simulink model "Simulacion"  (R2022a)
settings: Solver=VariableStepAuto  StartTime=0.0  StopTime=1  RelTol=1e-3
values from neighbouring files (symbols this model uses):
  Cbus = 80e-3    (= 0.08)    [Simulacion.m]
  D = 1e-3    (= 0.001)    [Simulacion.m]
  f = 50    [Simulacion.m]
  Fs = Vs*sqrt(2/3)/(2*pi*f)    [Simulacion.m]
  fsw = 4e3    (= 4000)    [Simulacion.m]
  J = 127    [Simulacion.m]
  ki_id = (wni^2)*Lr*sigma    (= 491.599501999)    [Simulacion.m]
  ki_idg = (wnig^2)*Lg    (= 56.8489213503)    [Simulacion.m]
  ki_iq = ki_id    (= 491.599501999)    [Simulacion.m]
  ki_iqg = ki_idg    (= 56.8489213503)    [Simulacion.m]
  ki_n = ((wnn^2)*J)/p    (= 25400)    [Simulacion.m]
  ki_v = -300000    [Simulacion.m]
  kp_id = (2*wni*sigma*Lr)-Rr    (= 0.5771)    [Simulacion.m]
  kp_idg = (2*wnig*Lg)-Rg    (= 0.301572894745)    [Simulacion.m]
  kp_iq = kp_id    (= 0.5771)    [Simulacion.m]
  kp_iqg = kp_idg    (= 0.301572894745)    [Simulacion.m]
  kp_n = (2*wnn*J)/p    (= 2540)    [Simulacion.m]
  kp_v = -1000    [Simulacion.m]
  Kpg = 1/(1.5*Vs*sqrt(2/3))    [Simulacion.m]
  Kqg = -Kpg    [Simulacion.m]
  Lg = 400e-6    (= 0.0004)    [Simulacion.m]
  Lm = 2.5e-3    (= 0.0025)    [Simulacion.m]
  Ls = Lm+Lsi    (= 0.002587)    [Simulacion.m]
  Lsi = 0.087e-3    (= 8.7e-05)    [Simulacion.m]
  p = 2    [Simulacion.m]
  Ps = 2e6    (= 2000000)    [Simulacion.m]
  Rg = 20e-6    (= 2e-05)    [Simulacion.m]
  Rr = 2.9e-3    (= 0.0029)    [Simulacion.m]
  Rs = 2.6e-3    (= 0.0026)    [Simulacion.m]
  Tem = 12732    [Simulacion.m]
  Ts = 1/fsw/50    (= 5e-06)    [Simulacion.m]
  Vbus = Vr_stator*sqrt(2)    [Simulacion.m]
  Vs = 690    [Simulacion.m]
undefined symbols (not defined in the file or in its folder): DiscIntNeverNeededParam
libraries: spsSeriesRLCBranchLib x4, spsThreePhaseVIMeasurementLib x3, spsPWMGenerator2LevelLib x2, spsUniversalBridgeLib x2, spsAsynchronousMachineSIUnitsLib x1, spsGroundLib x1, spsThreePhaseProgrammableVoltageSourceLib x1, spsThreePhaseTransformerTwoWindingsLib x1, spsVoltageMeasurementLib x1, spspowerguiLib x1
settings Model: Creator=ontib  LastModifiedBy=ontib

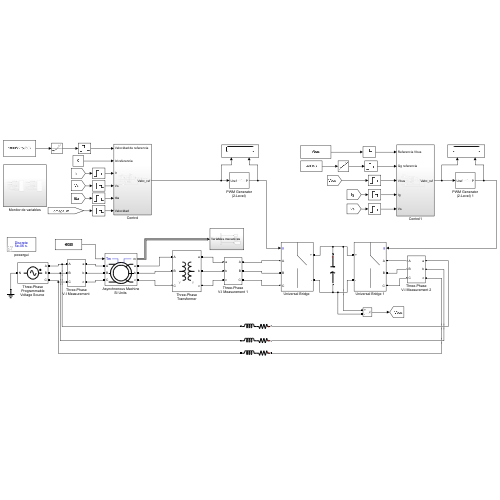
[thumbnail: Simulink's stored preview of the top-level diagram]
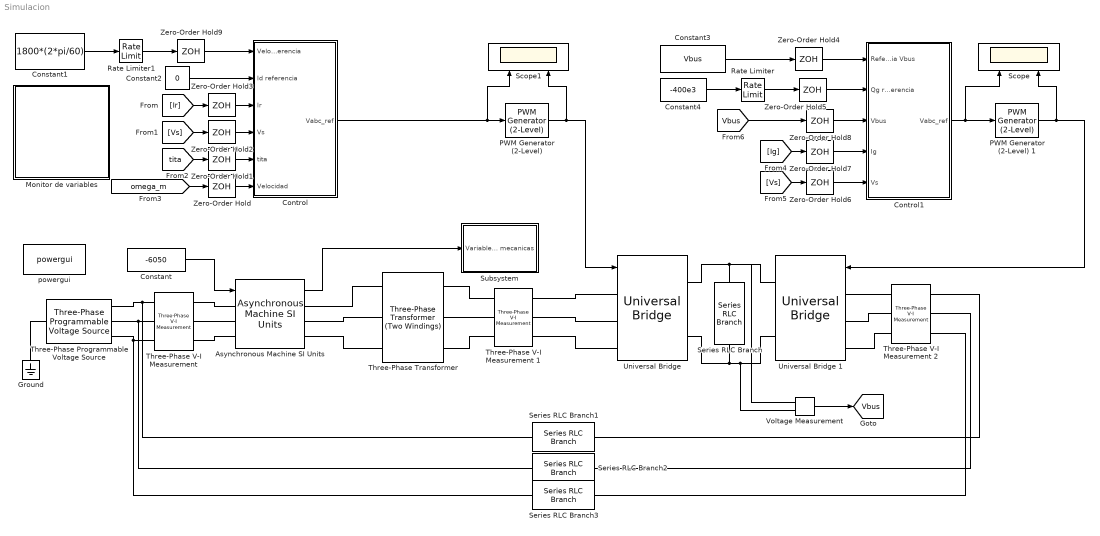
== system Simulacion ==
  "Asynchronous Machine SI Units " : spsAsynchronousMachineSIUnitsLib/Asynchronous Machine SI Units  RotorType=Wound  PresetModel=No  MechanicalLoad=Torque Tm  ShowDetailedParameters=on  ReferenceFrame=Rotor  Units=SI  MeasurementBus=off  NominalParameters=[Ps Vs f]  VoltageRatio=1  Stator=[Rs Ls]  Rotor=[Rr Lsi]  Cage1=[0.4155 0.002066]  Cage2=[0.4168 0.0003495]  Lm=Lm  Mechanical=[J D 2]  PolePairs=2  InitialConditions=[1 0 0 0 0 0 0 0]  SimulateSaturation=off  Saturation=[14.03593122, 27.81365428, 53.79336849, 72.68890987, 97.98006896, 148.6815601, 215.7428561, 302.9841135, 428.7778367 ; 230, 322, 414, 460, 506, 552, 598, 644, 690]  LoadFlowParameters=1492000  TsPowergui=0  TsBlock=-1  IterativeModel=Trapezoidal non iterative  IterativeDiscreteModel=Trapezoidal non iterative  Pmec=1.492e+006
  Constant : Constant  Value=-6050
  Constant1 : Constant  Value=1800*(2*pi/60)
  Constant2 : Constant  Value=0
  Constant3 : Constant  Value=Vbus
  Constant4 : Constant  Value=-400e3
  Control : Subsystem
  Control1 : Subsystem
  Ground : spsGroundLib/Ground  LConnTagsString=a
  Monitor de variables : Subsystem
  "PWM Generator (2-Level) " : spsPWMGenerator2LevelLib/PWM Generator (2-Level)  ModulatorType=Three-phase bridge (6 pulses)  ModulatorMode=Unsynchronized  Fc=fsw  Pc=0  nF=27  MinMax="[ -1  1 ]"  SamplingTechnique=Symmetrical regular (single edge)  ModulatingSignals=off  m=0.8  Freq=60  Phase=0  Ts=0  ShowCarrierOutport=off
  PWM Generator (2-Level) 1 : spsPWMGenerator2LevelLib/PWM Generator (2-Level)  ModulatorType=Three-phase bridge (6 pulses)  ModulatorMode=Unsynchronized  Fc=fsw  Pc=0  nF=27  MinMax="[ -1  1 ]"  SamplingTechnique=Symmetrical regular (single edge)  ModulatingSignals=off  m=0.8  Freq=60  Phase=0  Ts=0  ShowCarrierOutport=off
  Rate Limiter : RateLimiter  RisingSlewLimit=1000e3/2  FallingSlewLimit=-1000e3/2  SampleTimeMode=inherited
  Rate Limiter1 : RateLimiter  RisingSlewLimit=100  FallingSlewLimit=-100  SampleTimeMode=inherited
  Scope : Scope  NumInputPorts=2
  Scope1 : Scope  NumInputPorts=2
  Series RLC Branch : spsSeriesRLCBranchLib/Series RLC Branch  LConnTagsString=__new0  RConnTagsString=__new0  BranchType=C  Resistance=1  Inductance=1e-3  SetiL0=off  InitialCurrent=0  Capacitance=Cbus  Setx0=off  InitialVoltage=0  Measurements=Branch voltage
  Series RLC Branch1 : spsSeriesRLCBranchLib/Series RLC Branch  LConnTagsString=__new0  RConnTagsString=__new0  BranchType=RL  Resistance=Rg  Inductance=Lg  SetiL0=off  InitialCurrent=0  Capacitance=Cbus  Setx0=off  InitialVoltage=0  Measurements=Branch voltage
  Series RLC Branch2 : spsSeriesRLCBranchLib/Series RLC Branch  LConnTagsString=__new0  RConnTagsString=__new0  BranchType=RL  Resistance=Rg  Inductance=Lg  SetiL0=off  InitialCurrent=0  Capacitance=Cbus  Setx0=off  InitialVoltage=0  Measurements=Branch voltage
  Series RLC Branch3 : spsSeriesRLCBranchLib/Series RLC Branch  LConnTagsString=__new0  RConnTagsString=__new0  BranchType=RL  Resistance=Rg  Inductance=Lg  SetiL0=off  InitialCurrent=0  Capacitance=Cbus  Setx0=off  InitialVoltage=0  Measurements=Branch voltage
  Subsystem : Subsystem
  "Three-Phase Programmable Voltage Source " : spsThreePhaseProgrammableVoltageSourceLib/Three-Phase Programmable Voltage Source  PositiveSequence="[Vs  0 f]"  VariationEntity=None  VariationType=Table of time-amplitude pairs  VariationTypeAlt=Step  VariationStep=0.5  VariationRate=10  VariationMagnitude=0.3  VariationFrequency=2  VariationTiming=[1 2]  VariationPhaseA=off  Amplitudes=[1 0.8 1.2 1.0]  TimeValues=[0 0.1 0.15 0.2]  HarmonicGeneration=off  HarmonicA=[3 0.2 -25 0]  HarmonicB=[2 0.15 35 2]  Timing="[0.05  3]"  BusType=swing  Pref=0  Qref=0  Qmin=-inf  Qmax=inf
  Three-Phase Transformer : spsThreePhaseTransformerTwoWindingsLib/Three-Phase Transformer (Two Windings)  Winding1Connection=Y  Winding2Connection=Y  CoreType=Three single-phase transformers  SetSaturation=off  Hysteresis=off  DataFile='hysteresis'  SetInitialFlux=off  Measurements=None  UNITS=SI  NominalPower=[ Ps , f ]  Winding1=[Vs 0 0]  Winding2=[Vs/u 0 0]  Rm=1.0804e+06  Lm=3439.2  L0=0.5  Saturation=[0 0;0.66653 2292.3;277.72 2903.6]  InitialFluxes=[ 0.8 , -0.8 , 0.7 ]  BreakLoop=off  DiscreteSolver=Trapezoidal iterative  DataType=on  TransfoNumber=1
  "Three-Phase V-I Measurement " : spsThreePhaseVIMeasurementLib/Three-Phase V-I Measurement  VoltageMeasurement=phase-to-ground  SetLabelV=on  LabelV=Vs  Vpu=off  VpuLL=off  CurrentMeasurement=yes  SetLabelI=on  LabelI=Is  Ipu=off  Pbase=100e6  Vbase=500e3  OutputType=Complex  PhasorSimulation=off  PSBequivalent=0
  Three-Phase V-I Measurement 1 : spsThreePhaseVIMeasurementLib/Three-Phase V-I Measurement  VoltageMeasurement=no  SetLabelV=off  LabelV=Vs  Vpu=off  VpuLL=off  CurrentMeasurement=yes  SetLabelI=on  LabelI=Ir  Ipu=off  Pbase=100e6  Vbase=500e3  OutputType=Complex  PhasorSimulation=off  PSBequivalent=0
  Three-Phase V-I Measurement 2 : spsThreePhaseVIMeasurementLib/Three-Phase V-I Measurement  VoltageMeasurement=no  SetLabelV=off  LabelV=Vs  Vpu=off  VpuLL=off  CurrentMeasurement=yes  SetLabelI=on  LabelI=Ig  Ipu=off  Pbase=100e6  Vbase=500e3  OutputType=Complex  PhasorSimulation=off  PSBequivalent=0
  "Universal Bridge " : spsUniversalBridgeLib/Universal Bridge  Arms=3  SnubberResistance=1e5  SnubberCapacitance=inf  Device=Ideal Switches  Ron=1e-3  Lon=0  ForwardVoltages="[  0  0  ]"  ForwardVoltage=0  GTOparameters=[ 10e-6 , 20e-6 ]  IGBTparameters=[ 1e-6 , 2e-6 ]  Measurements=None  Measurements_2=None  converterType=Rectifier
  Universal Bridge 1 : spsUniversalBridgeLib/Universal Bridge  Arms=3  SnubberResistance=1e5  SnubberCapacitance=inf  Device=Ideal Switches  Ron=1e-3  Lon=0  ForwardVoltages="[  0  0  ]"  ForwardVoltage=0  GTOparameters=[ 10e-6 , 20e-6 ]  IGBTparameters=[ 1e-6 , 2e-6 ]  Measurements=None  Measurements_2=None  converterType=Rectifier
  Voltage Measurement : spsVoltageMeasurementLib/Voltage Measurement  PhasorSimulation=off  OutputType=Complex  PSBequivalent=0
  Zero-Order Hold{,1..9} (10 alike) : ZeroOrderHold  SampleTime=1/fsw
  powergui : spspowerguiLib/powergui  Priority=1  SimulationMode=Discrete  SampleTime=Ts  frequency=60  Iterations=50  frequencyindice=50  Pbase=100e6  ErrMax=1e-4  UnitsV=kV  UnitsW=MW  buscounter=0  FunctionMessages=off  echomessages=off  EnableUseOfTLC=off  CurrentSourceSwitches=off  DisableSnubberDevices=off  DisableRonSwitches=off  DisableVfSwitches=off  DisplayEquations=off  AutomaticDiscreteSolvers=off  SolverType=Tustin/Backward Euler (TBE)  Interpol=off  ExternalGateDelay=off  methode=off  Ts=100  x0status=blocks  SPID=on  SwTol=0  HookPort=off  NonlinearTolerance=1e-4  nMaxIteration=100  ContinueOnMaxIteration=off  RestoreLinks=warning  ResistiveCurrentMeasurement=off  Frange=[0:2:500]  Ylog=off  Xlog=on  ShowGrid=off  save=off  variable=ZData  structure=0  ZoomFFT=off  StartTime=0.0  cycles=1  DisplayStyle=1  fundamental=60  FreqAxis=off  MaxFrequency=1000  frequencyindicesteady=1  RmsSteady=1  display=off
  tag scope: Vbus=global
  wires:
  "PWM Generator (2-Level) "/1 -> "Universal Bridge "/1, Scope1/2
  Control/1(Vabc_ref) -> Scope1/1, "PWM Generator (2-Level) "/1
  [Ir] -> Zero-Order Hold3/1
  [Vs] -> Zero-Order Hold2/1
  Constant2/1 -> Control/2(Id referencia)
  Zero-Order Hold9/1 -> Control/1(Velocidad de referencia)
  "Asynchronous Machine SI Units "/1 -> Subsystem/1(Variables mecanicas)
  [tita] -> Zero-Order Hold1/1
  [omega_m] -> Zero-Order Hold/1
  Constant/1 -> "Asynchronous Machine SI Units "/1
  Zero-Order Hold/1 -> Control/6(Velocidad)
  Zero-Order Hold1/1 -> Control/5(tita)
  Zero-Order Hold2/1 -> Control/4(Vs)
  Zero-Order Hold3/1 -> Control/3(Ir)
  PWM Generator (2-Level) 1/1 -> Universal Bridge 1/1, Scope/2
  Zero-Order Hold7/1 -> Control1/4(Ig)
  Zero-Order Hold6/1 -> Control1/5(Vs)
  [Ig] -> Zero-Order Hold7/1
  Constant4/1 -> Rate Limiter/1
  [Vs] -> Zero-Order Hold6/1
  Control1/1(Vabc_ref) -> Scope/1, PWM Generator (2-Level) 1/1
  Constant3/1 -> Zero-Order Hold4/1
  Zero-Order Hold4/1 -> Control1/1(Referencia Vbus)
  Rate Limiter/1 -> Zero-Order Hold5/1
  Zero-Order Hold5/1 -> Control1/2(Qg referencia)
  Voltage Measurement/1 -> [Vbus]
  [Vbus] -> Zero-Order Hold8/1
  Zero-Order Hold8/1 -> Control1/3(Vbus)
  Constant1/1 -> Rate Limiter1/1
  Rate Limiter1/1 -> Zero-Order Hold9/1
  connections:
  Ground/LConn1 -- "Three-Phase Programmable Voltage Source "/LConn1
  "Three-Phase V-I Measurement "/RConn1 -- "Asynchronous Machine SI Units "/LConn1
  "Asynchronous Machine SI Units "/LConn2 -- "Three-Phase V-I Measurement "/RConn2
  "Three-Phase V-I Measurement "/RConn3 -- "Asynchronous Machine SI Units "/LConn3
  "Three-Phase V-I Measurement "/LConn1 -- Series RLC Branch1/RConn1 -- "Three-Phase Programmable Voltage Source "/RConn1
  "Three-Phase V-I Measurement "/LConn2 -- Series RLC Branch2/RConn1 -- "Three-Phase Programmable Voltage Source "/RConn2
  "Three-Phase V-I Measurement "/LConn3 -- Series RLC Branch3/RConn1 -- "Three-Phase Programmable Voltage Source "/RConn3
  Three-Phase V-I Measurement 1/LConn1 -- "Universal Bridge "/LConn1
  Three-Phase V-I Measurement 1/LConn2 -- "Universal Bridge "/LConn2
  Three-Phase V-I Measurement 1/LConn3 -- "Universal Bridge "/LConn3
  Series RLC Branch/LConn1 -- Voltage Measurement/LConn1 -- Universal Bridge 1/RConn1 -- "Universal Bridge "/RConn1
  Universal Bridge 1/RConn2 -- Voltage Measurement/LConn2 -- "Universal Bridge "/RConn2 -- Series RLC Branch/RConn1
  Three-Phase V-I Measurement 2/LConn1 -- Universal Bridge 1/LConn1
  Three-Phase V-I Measurement 2/LConn2 -- Universal Bridge 1/LConn2
  Three-Phase V-I Measurement 2/LConn3 -- Universal Bridge 1/LConn3
  Series RLC Branch1/LConn1 -- Three-Phase V-I Measurement 2/RConn1
  Series RLC Branch2/LConn1 -- Three-Phase V-I Measurement 2/RConn2
  Series RLC Branch3/LConn1 -- Three-Phase V-I Measurement 2/RConn3
  Three-Phase Transformer/RConn1 -- Three-Phase V-I Measurement 1/RConn1
  Three-Phase V-I Measurement 1/RConn2 -- Three-Phase Transformer/RConn2
  Three-Phase V-I Measurement 1/RConn3 -- Three-Phase Transformer/RConn3
  Three-Phase Transformer/LConn1 -- "Asynchronous Machine SI Units "/RConn1
  Three-Phase Transformer/LConn2 -- "Asynchronous Machine SI Units "/RConn2
  "Asynchronous Machine SI Units "/RConn3 -- Three-Phase Transformer/LConn3

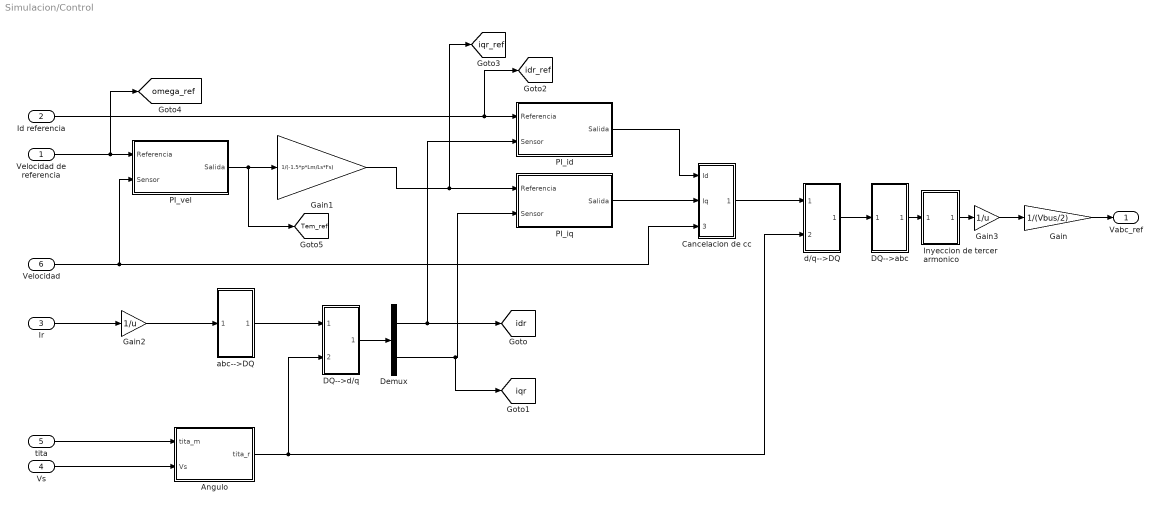
== system Simulacion/Control ==
  Velocidad de referencia : Inport
  Id referencia : Inport  Port=2
  Ir : Inport  Port=3
  Vs : Inport  Port=4
  tita : Inport  Port=5
  Velocidad : Inport  Port=6
  Angulo : Subsystem
  Cancelacion de cc : Subsystem
  DQ-->abc : Subsystem
  DQ-->d/q : Subsystem
  Demux : Demux  Outputs=2
  Gain : Gain  Gain=1/(Vbus/2)
  Gain1 : Gain  Gain=1/(-1.5*p*Lm/Ls*Fs)
  Gain2 : Gain  Gain=1/u
  Gain3 : Gain  Gain=1/u
  Inyeccion de tercer armonico : Subsystem
  PI_id : Subsystem
  PI_iq : Subsystem
  PI_vel : Subsystem
  abc-->DQ : Subsystem
  d/q-->DQ : Subsystem
  Vabc_ref : Outport
  tag scope: Tem_ref=global, idr=global, idr_ref=global, iqr=global, iqr_ref=global, omega_ref=global
  wires:
  Gain/1 -> Vabc_ref/1
  d/q-->DQ/1(DQ) -> DQ-->abc/1(D/Q)
  abc-->DQ/1(D/Q) -> DQ-->d/q/1(D/Q)
  Ir/1 -> Gain2/1
  DQ-->abc/1(abc) -> Inyeccion de tercer armonico/1(abc)
  Inyeccion de tercer armonico/1(Out1) -> Gain3/1
  tita/1 -> Angulo/1(tita_m)
  Vs/1 -> Angulo/2(Vs)
  Angulo/1(tita_r) -> DQ-->d/q/2(tita), d/q-->DQ/2(tita)
  Cancelacion de cc/1(d/q) -> d/q-->DQ/1(d/q)
  PI_iq/1(Salida) -> Cancelacion de cc/2(Iq)
  PI_id/1(Salida) -> Cancelacion de cc/1(Id)
  Velocidad/1 -> PI_vel/2(Sensor), Cancelacion de cc/3(omega)
  DQ-->d/q/1(d/q) -> Demux/1
  Demux/2 -> [iqr], PI_iq/2(Sensor)
  Demux/1 -> [idr], PI_id/2(Sensor)
  Velocidad de referencia/1 -> [omega_ref], PI_vel/1(Referencia)
  PI_vel/1(Salida) -> [Tem_ref], Gain1/1
  Gain1/1 -> [iqr_ref], PI_iq/1(Referencia)
  Id referencia/1 -> [idr_ref], PI_id/1(Referencia)
  Gain3/1 -> Gain/1
  Gain2/1 -> abc-->DQ/1(abc)

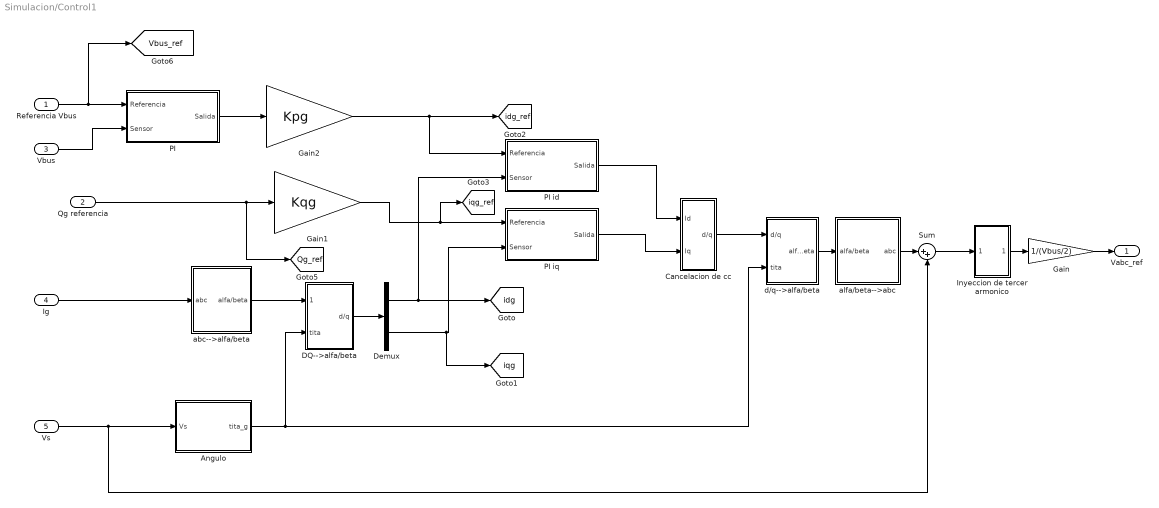
== system Simulacion/Control1 ==
  Referencia Vbus : Inport
  Qg referencia : Inport  Port=2
  Vbus : Inport  Port=3
  Ig : Inport  Port=4
  Vs : Inport  Port=5
  Angulo : Subsystem
  Cancelacion de cc : Subsystem
  DQ-->alfa/beta : Subsystem
  Demux : Demux  Outputs=2
  Gain : Gain  Gain=1/(Vbus/2)
  Gain1 : Gain  Gain=Kqg
  Gain2 : Gain  Gain=Kpg
  Inyeccion de tercer armonico : Subsystem
  PI : Subsystem
  PI id : Subsystem
  PI iq : Subsystem
  Sum : Sum  Inputs=|++
  abc-->alfa/beta : Subsystem
  alfa/beta-->abc : Subsystem
  d/q-->alfa/beta : Subsystem
  Vabc_ref : Outport
  tag scope: Qg_ref=global, Vbus_ref=global, idg=global, idg_ref=global, iqg=global, iqg_ref=global
  wires:
  Gain/1 -> Vabc_ref/1
  d/q-->alfa/beta/1(alfa/beta) -> alfa/beta-->abc/1(alfa/beta)
  abc-->alfa/beta/1(alfa/beta) -> DQ-->alfa/beta/1(alfa/beta)
  Ig/1 -> abc-->alfa/beta/1(abc)
  Inyeccion de tercer armonico/1(Out1) -> Gain/1
  Vs/1 -> Sum/2, Angulo/1(Vs)
  Angulo/1(tita_g) -> d/q-->alfa/beta/2(tita), DQ-->alfa/beta/2(tita)
  Cancelacion de cc/1(d/q) -> d/q-->alfa/beta/1(d/q)
  PI iq/1(Salida) -> Cancelacion de cc/2(Iq)
  PI id/1(Salida) -> Cancelacion de cc/1(Id)
  DQ-->alfa/beta/1(d/q) -> Demux/1
  Demux/2 -> [iqg], PI iq/2(Sensor)
  Demux/1 -> [idg], PI id/2(Sensor)
  Qg referencia/1 -> [Qg_ref], Gain1/1
  Gain1/1 -> [iqg_ref], PI iq/1(Referencia)
  PI/1(Salida) -> Gain2/1
  Gain2/1 -> [idg_ref], PI id/1(Referencia)
  Referencia Vbus/1 -> [Vbus_ref], PI/1(Referencia)
  Vbus/1 -> PI/2(Sensor)
  alfa/beta-->abc/1(abc) -> Sum/1
  Sum/1 -> Inyeccion de tercer armonico/1(abc)

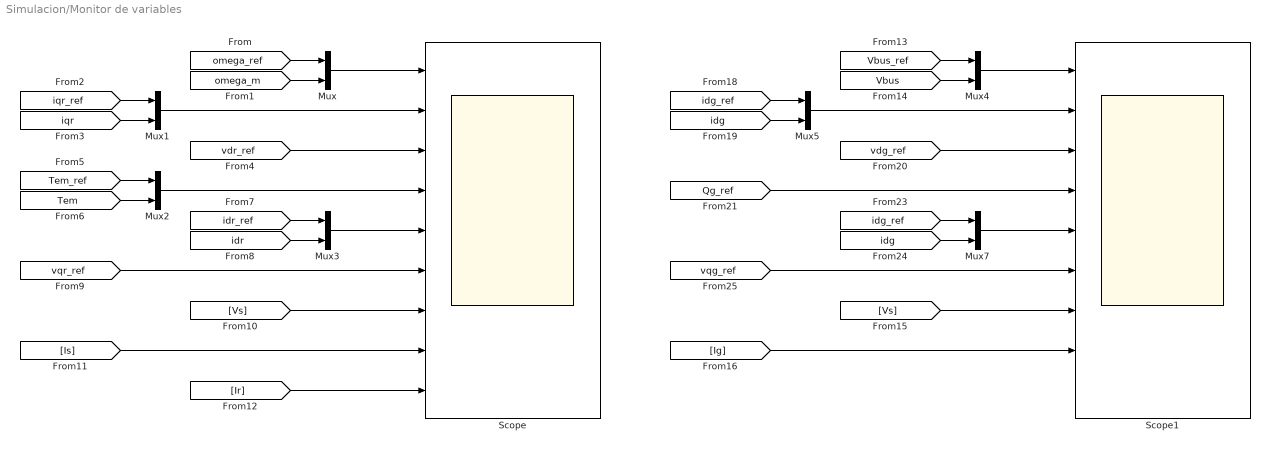
== system Simulacion/Monitor de variables ==
  Mux{,1..5,7} (7 alike) : Mux  Inputs=2
  Scope : Scope  NumInputPorts=9
  Scope1 : Scope  NumInputPorts=9
  wires:
  [omega_ref] -> Mux/1
  [omega_m] -> Mux/2
  [iqr_ref] -> Mux1/1
  [iqr] -> Mux1/2
  Mux/1 -> Scope/1
  Mux1/1 -> Scope/2
  [vdr_ref] -> Scope/3
  Mux2/1 -> Scope/4
  [Tem_ref] -> Mux2/1
  [Tem] -> Mux2/2
  [idr_ref] -> Mux3/1
  [idr] -> Mux3/2
  Mux3/1 -> Scope/5
  [vqr_ref] -> Scope/6
  [Vs] -> Scope/7
  [Ir] -> Scope/9
  [Is] -> Scope/8
  [idg] -> Mux7/2
  Mux7/1 -> Scope1/5
  [Ig] -> Scope1/8
  [Vbus_ref] -> Mux4/1
  [Vbus] -> Mux4/2
  [idg_ref] -> Mux7/1
  [vqg_ref] -> Scope1/6
  Mux4/1 -> Scope1/1
  Mux5/1 -> Scope1/2
  [vdg_ref] -> Scope1/3
  [idg] -> Mux5/2
  [idg_ref] -> Mux5/1
  [Vs] -> Scope1/7
  [Qg_ref] -> Scope1/4

== system Simulacion/Subsystem ==
  Variables mecanicas : Inport
  Bus Selector : BusSelector  OutputSignals=Mechanical.Rotor angle thetam (rad),Mechanical.Electromagnetic torque Te (N*m),Mechanical.Rotor speed (wm)
  tag scope: Tem=global, omega_m=global, tita=global
  wires:
  Bus Selector/1 -> [tita]  "<Rotor angle thetam (rad)>"
  Variables mecanicas/1 -> Bus Selector/1
  Bus Selector/2 -> [Tem]  "<Electromagnetic torque Te (N*m)>"
  Bus Selector/3 -> [omega_m]  "<Rotor speed (wm)>"

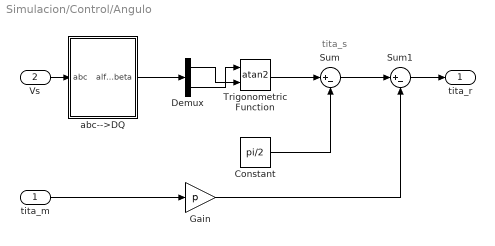
== system Simulacion/Control/Angulo ==
  note: tita_s
  tita_m : Inport
  Vs : Inport  Port=2
  Constant : Constant  Value=pi/2
  Demux : Demux  Outputs=2
  Gain : Gain  Gain=p
  Sum : Sum  Inputs=|+-
  Sum1 : Sum  Inputs=|+-
  "Trigonometric Function " : Trigonometry  Operator=atan2
  abc-->DQ : Subsystem
  tita_r : Outport
  wires:
  Vs/1 -> abc-->DQ/1(abc)
  abc-->DQ/1(alfa/beta) -> Demux/1
  Demux/1 -> "Trigonometric Function "/2
  Demux/2 -> "Trigonometric Function "/1
  "Trigonometric Function "/1 -> Sum/1
  Constant/1 -> Sum/2
  Sum/1 -> Sum1/1
  Sum1/1 -> tita_r/1
  tita_m/1 -> Gain/1
  Gain/1 -> Sum1/2

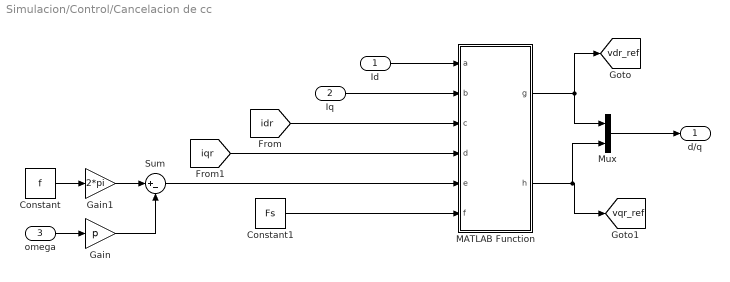
== system Simulacion/Control/Cancelacion de cc ==
  Id : Inport
  Iq : Inport  Port=2
  omega : Inport  Port=3
  Constant : Constant  Value=f
  Constant1 : Constant  Value=Fs
  Gain : Gain  Gain=p
  Gain1 : Gain  Gain=2*pi
  MATLAB Function : MATLAB Function  TreatAsAtomicUnit=on
  Mux : Mux  Inputs=2
  Sum : Sum  Inputs=|+-
  d/q : Outport
  tag scope: vdr_ref=global, vqr_ref=global
  wires:
  Mux/1 -> d/q/1
  MATLAB Function/1(g) -> Mux/1, [vdr_ref]
  MATLAB Function/2(h) -> Mux/2, [vqr_ref]
  Id/1 -> MATLAB Function/1(a)
  Iq/1 -> MATLAB Function/2(b)
  [idr] -> MATLAB Function/3(c)
  [iqr] -> MATLAB Function/4(d)
  Sum/1 -> MATLAB Function/5(e)
  Gain/1 -> Sum/2
  Gain1/1 -> Sum/1
  omega/1 -> Gain/1
  Constant/1 -> Gain1/1
  Constant1/1 -> MATLAB Function/6(f)

== system Simulacion/Control/DQ-->abc ==
  D/Q : Inport
  Demux : Demux  Outputs=2
  MATLAB Function : MATLAB Function  TreatAsAtomicUnit=on
  Mux : Mux  Inputs=3
  abc : Outport
  wires:
  MATLAB Function/1(d) -> Mux/1
  MATLAB Function/2(e) -> Mux/2
  MATLAB Function/3(f) -> Mux/3
  Mux/1 -> abc/1
  Demux/1 -> MATLAB Function/1(a)
  D/Q/1 -> Demux/1
  Demux/2 -> MATLAB Function/2(b)

== system Simulacion/Control/DQ-->d//q ==
  D/Q : Inport
  tita : Inport  Port=2
  Demux : Demux  Outputs=2
  MATLAB Function : MATLAB Function  TreatAsAtomicUnit=on
  Mux : Mux  Inputs=2
  d/q : Outport
  wires:
  MATLAB Function/1(d) -> Mux/1
  MATLAB Function/2(e) -> Mux/2
  tita/1 -> MATLAB Function/3(c)
  D/Q/1 -> Demux/1
  Demux/1 -> MATLAB Function/1(a)
  Demux/2 -> MATLAB Function/2(b)
  Mux/1 -> d/q/1

== system Simulacion/Control/Inyeccion de tercer armonico ==
  abc : Inport
  Gain : Gain  Gain=-0.5
  Max : MinMax  Function=max
  Min : MinMax
  Sum : Sum  Inputs=|++
  Sum1 : Sum  Inputs=|++
  Out1 : Outport
  wires:
  abc/1 -> Max/1, Min/1, Sum/1
  Sum/1 -> Out1/1
  Min/1 -> Sum1/1
  Sum1/1 -> Gain/1
  Gain/1 -> Sum/2
  Max/1 -> Sum1/2

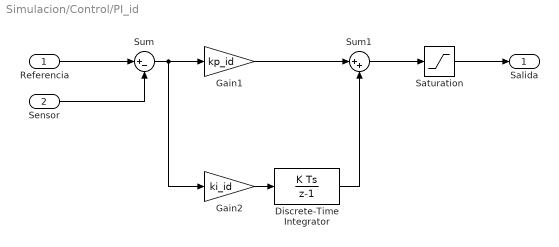
== system Simulacion/Control/PI_id ==
  Referencia : Inport
  Sensor : Inport  Port=2
  Discrete-Time Integrator : DiscreteIntegrator  SampleTime=1/fsw  LimitOutput=on  UpperSaturationLimit=Vbus/sqrt(3)  LowerSaturationLimit=-Vbus/sqrt(3)  ICPrevOutput=DiscIntNeverNeededParam  ICPrevScaledInput=DiscIntNeverNeededParam
  Gain1 : Gain  Gain=kp_id
  Gain2 : Gain  Gain=ki_id
  Saturation : Saturate  UpperLimit=Vbus/sqrt(3)  LowerLimit=-Vbus/sqrt(3)
  Sum : Sum  Inputs=|+-
  Sum1 : Sum  Inputs=|++
  Salida : Outport
  wires:
  Sum/1 -> Gain2/1, Gain1/1
  Referencia/1 -> Sum/1
  Sensor/1 -> Sum/2
  Gain1/1 -> Sum1/1
  Sum1/1 -> Saturation/1
  Saturation/1 -> Salida/1
  Gain2/1 -> Discrete-Time Integrator/1
  Discrete-Time Integrator/1 -> Sum1/2

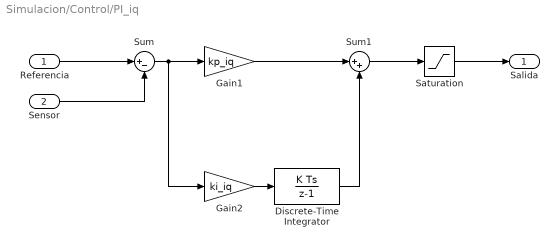
== system Simulacion/Control/PI_iq ==
  Referencia : Inport
  Sensor : Inport  Port=2
  Discrete-Time Integrator : DiscreteIntegrator  SampleTime=1/fsw  LimitOutput=on  UpperSaturationLimit=Vbus/sqrt(3)  LowerSaturationLimit=-Vbus/sqrt(3)  ICPrevOutput=DiscIntNeverNeededParam  ICPrevScaledInput=DiscIntNeverNeededParam
  Gain1 : Gain  Gain=kp_iq
  Gain2 : Gain  Gain=ki_iq
  Saturation : Saturate  UpperLimit=Vbus/sqrt(3)  LowerLimit=-Vbus/sqrt(3)
  Sum : Sum  Inputs=|+-
  Sum1 : Sum  Inputs=|++
  Salida : Outport
  wires:
  Sum/1 -> Gain2/1, Gain1/1
  Referencia/1 -> Sum/1
  Sensor/1 -> Sum/2
  Gain1/1 -> Sum1/1
  Sum1/1 -> Saturation/1
  Saturation/1 -> Salida/1
  Gain2/1 -> Discrete-Time Integrator/1
  Discrete-Time Integrator/1 -> Sum1/2

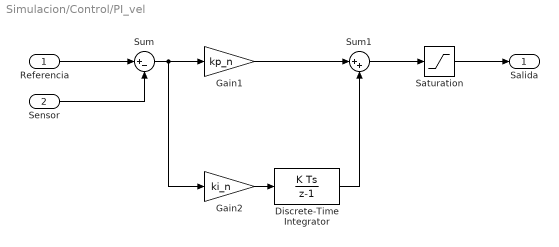
== system Simulacion/Control/PI_vel ==
  Referencia : Inport
  Sensor : Inport  Port=2
  Discrete-Time Integrator : DiscreteIntegrator  SampleTime=1/fsw  LimitOutput=on  UpperSaturationLimit=Tem  LowerSaturationLimit=-Tem  ICPrevOutput=DiscIntNeverNeededParam  ICPrevScaledInput=DiscIntNeverNeededParam
  Gain1 : Gain  Gain=kp_n
  Gain2 : Gain  Gain=ki_n
  Saturation : Saturate  UpperLimit=Tem  LowerLimit=-Tem
  Sum : Sum  Inputs=|+-
  Sum1 : Sum  Inputs=|++
  Salida : Outport
  wires:
  Sum/1 -> Gain2/1, Gain1/1
  Referencia/1 -> Sum/1
  Sensor/1 -> Sum/2
  Gain1/1 -> Sum1/1
  Sum1/1 -> Saturation/1
  Saturation/1 -> Salida/1
  Gain2/1 -> Discrete-Time Integrator/1
  Discrete-Time Integrator/1 -> Sum1/2

== system Simulacion/Control/abc-->DQ ==
  abc : Inport
  Demux : Demux  Outputs=3
  MATLAB Function : MATLAB Function  TreatAsAtomicUnit=on
  Mux : Mux  Inputs=2
  D/Q : Outport
  wires:
  abc/1 -> Demux/1
  Demux/2 -> MATLAB Function/2(b)
  Demux/1 -> MATLAB Function/1(a)
  MATLAB Function/1(d) -> Mux/1
  MATLAB Function/2(e) -> Mux/2
  Mux/1 -> D/Q/1
  Demux/3 -> MATLAB Function/3(c)

== system Simulacion/Control/d//q-->DQ ==
  d/q : Inport
  tita : Inport  Port=2
  Demux : Demux  Outputs=2
  MATLAB Function : MATLAB Function  TreatAsAtomicUnit=on
  Mux : Mux  Inputs=2
  DQ : Outport
  wires:
  Demux/1 -> MATLAB Function/1(a)
  d/q/1 -> Demux/1
  MATLAB Function/1(d) -> Mux/1
  tita/1 -> MATLAB Function/3(c)
  Demux/2 -> MATLAB Function/2(b)
  MATLAB Function/2(e) -> Mux/2
  Mux/1 -> DQ/1

== system Simulacion/Control1/Angulo ==
  Vs : Inport
  Demux : Demux  Outputs=2
  "Trigonometric Function " : Trigonometry  Operator=atan2
  abc-->alfa/beta : Subsystem
  tita_g : Outport
  wires:
  Vs/1 -> abc-->alfa/beta/1(abc)
  abc-->alfa/beta/1(alfa/beta) -> Demux/1
  Demux/1 -> "Trigonometric Function "/2
  Demux/2 -> "Trigonometric Function "/1
  "Trigonometric Function "/1 -> tita_g/1

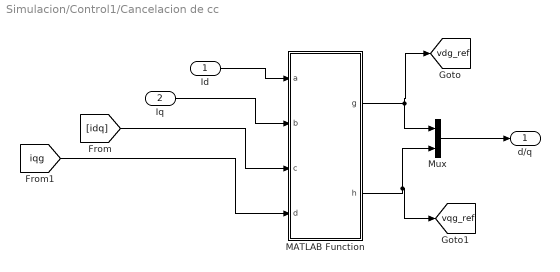
== system Simulacion/Control1/Cancelacion de cc ==
  Id : Inport
  Iq : Inport  Port=2
  MATLAB Function : MATLAB Function  TreatAsAtomicUnit=on
  Mux : Mux  Inputs=2
  d/q : Outport
  tag scope: vdg_ref=global, vqg_ref=global
  wires:
  Mux/1 -> d/q/1
  MATLAB Function/1(g) -> [vdg_ref], Mux/1
  MATLAB Function/2(h) -> Mux/2, [vqg_ref]
  Id/1 -> MATLAB Function/1(a)
  Iq/1 -> MATLAB Function/2(b)
  [idq] -> MATLAB Function/3(c)
  [iqg] -> MATLAB Function/4(d)

== system Simulacion/Control1/DQ-->alfa//beta ==
  alfa/beta : Inport
  tita : Inport  Port=2
  Demux : Demux  Outputs=2
  MATLAB Function : MATLAB Function  TreatAsAtomicUnit=on
  Mux : Mux  Inputs=2
  d/q : Outport
  wires:
  MATLAB Function/1(d) -> Mux/1
  MATLAB Function/2(e) -> Mux/2
  tita/1 -> MATLAB Function/3(c)
  alfa/beta/1 -> Demux/1
  Demux/1 -> MATLAB Function/1(a)
  Demux/2 -> MATLAB Function/2(b)
  Mux/1 -> d/q/1

== system Simulacion/Control1/Inyeccion de tercer armonico ==
  abc : Inport
  Gain : Gain  Gain=-0.5
  Max : MinMax  Function=max
  Min : MinMax
  Sum : Sum  Inputs=|++
  Sum1 : Sum  Inputs=|++
  Out1 : Outport
  wires:
  abc/1 -> Max/1, Min/1, Sum/1
  Sum/1 -> Out1/1
  Min/1 -> Sum1/1
  Sum1/1 -> Gain/1
  Gain/1 -> Sum/2
  Max/1 -> Sum1/2

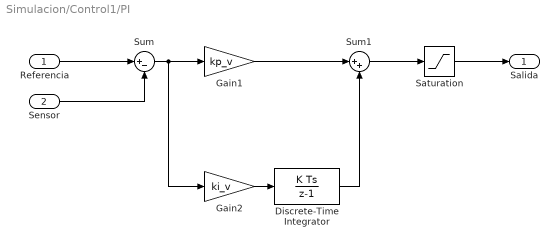
== system Simulacion/Control1/PI ==
  Referencia : Inport
  Sensor : Inport  Port=2
  Discrete-Time Integrator : DiscreteIntegrator  SampleTime=1/fsw  LimitOutput=on  UpperSaturationLimit=Ps*1/3  LowerSaturationLimit=-Ps*1/3  ICPrevOutput=DiscIntNeverNeededParam  ICPrevScaledInput=DiscIntNeverNeededParam
  Gain1 : Gain  Gain=kp_v
  Gain2 : Gain  Gain=ki_v
  Saturation : Saturate  UpperLimit=Ps*1/3  LowerLimit=-Ps*1/3
  Sum : Sum  Inputs=|+-
  Sum1 : Sum  Inputs=|++
  Salida : Outport
  wires:
  Sum/1 -> Gain2/1, Gain1/1
  Referencia/1 -> Sum/1
  Sensor/1 -> Sum/2
  Gain1/1 -> Sum1/1
  Sum1/1 -> Saturation/1
  Saturation/1 -> Salida/1
  Gain2/1 -> Discrete-Time Integrator/1
  Discrete-Time Integrator/1 -> Sum1/2

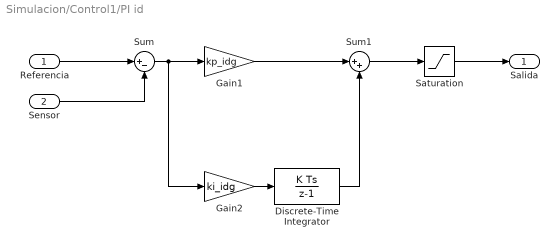
== system Simulacion/Control1/PI id ==
  Referencia : Inport
  Sensor : Inport  Port=2
  Discrete-Time Integrator : DiscreteIntegrator  SampleTime=1/fsw  LimitOutput=on  UpperSaturationLimit=Vbus/sqrt(3)  LowerSaturationLimit=-Vbus/sqrt(3)  ICPrevOutput=DiscIntNeverNeededParam  ICPrevScaledInput=DiscIntNeverNeededParam
  Gain1 : Gain  Gain=kp_idg
  Gain2 : Gain  Gain=ki_idg
  Saturation : Saturate  UpperLimit=Vbus/sqrt(3)  LowerLimit=-Vbus/sqrt(3)
  Sum : Sum  Inputs=|+-
  Sum1 : Sum  Inputs=|++
  Salida : Outport
  wires:
  Sum/1 -> Gain2/1, Gain1/1
  Referencia/1 -> Sum/1
  Sensor/1 -> Sum/2
  Gain1/1 -> Sum1/1
  Sum1/1 -> Saturation/1
  Saturation/1 -> Salida/1
  Gain2/1 -> Discrete-Time Integrator/1
  Discrete-Time Integrator/1 -> Sum1/2

== system Simulacion/Control1/PI iq ==
  Referencia : Inport
  Sensor : Inport  Port=2
  Discrete-Time Integrator : DiscreteIntegrator  SampleTime=1/fsw  LimitOutput=on  UpperSaturationLimit=Vbus/sqrt(3)  LowerSaturationLimit=-Vbus/sqrt(3)  ICPrevOutput=DiscIntNeverNeededParam  ICPrevScaledInput=DiscIntNeverNeededParam
  Gain1 : Gain  Gain=kp_iqg
  Gain2 : Gain  Gain=ki_iqg
  Saturation : Saturate  UpperLimit=Vbus/sqrt(3)  LowerLimit=-Vbus/sqrt(3)
  Sum : Sum  Inputs=|+-
  Sum1 : Sum  Inputs=|++
  Salida : Outport
  wires:
  Sum/1 -> Gain2/1, Gain1/1
  Referencia/1 -> Sum/1
  Sensor/1 -> Sum/2
  Gain1/1 -> Sum1/1
  Sum1/1 -> Saturation/1
  Saturation/1 -> Salida/1
  Gain2/1 -> Discrete-Time Integrator/1
  Discrete-Time Integrator/1 -> Sum1/2

== system Simulacion/Control1/abc-->alfa//beta ==
  abc : Inport
  Demux : Demux  Outputs=3
  MATLAB Function : MATLAB Function  TreatAsAtomicUnit=on
  Mux : Mux  Inputs=2
  alfa/beta : Outport
  wires:
  abc/1 -> Demux/1
  Demux/2 -> MATLAB Function/2(b)
  Demux/1 -> MATLAB Function/1(a)
  MATLAB Function/1(d) -> Mux/1
  MATLAB Function/2(e) -> Mux/2
  Mux/1 -> alfa/beta/1
  Demux/3 -> MATLAB Function/3(c)

== system Simulacion/Control1/alfa//beta-->abc ==
  alfa/beta : Inport
  Demux : Demux  Outputs=2
  MATLAB Function : MATLAB Function  TreatAsAtomicUnit=on
  Mux : Mux  Inputs=3
  abc : Outport
  wires:
  MATLAB Function/1(d) -> Mux/1
  MATLAB Function/2(e) -> Mux/2
  MATLAB Function/3(f) -> Mux/3
  Mux/1 -> abc/1
  Demux/1 -> MATLAB Function/1(a)
  alfa/beta/1 -> Demux/1
  Demux/2 -> MATLAB Function/2(b)

== system Simulacion/Control1/d//q-->alfa//beta ==
  d/q : Inport
  tita : Inport  Port=2
  Demux : Demux  Outputs=2
  MATLAB Function : MATLAB Function  TreatAsAtomicUnit=on
  Mux : Mux  Inputs=2
  alfa/beta : Outport
  wires:
  Demux/1 -> MATLAB Function/1(a)
  d/q/1 -> Demux/1
  MATLAB Function/1(d) -> Mux/1
  tita/1 -> MATLAB Function/3(c)
  Demux/2 -> MATLAB Function/2(b)
  MATLAB Function/2(e) -> Mux/2
  Mux/1 -> alfa/beta/1

== system Simulacion/Control/Angulo/abc-->DQ ==
  abc : Inport
  Demux : Demux  Outputs=3
  MATLAB Function : MATLAB Function  TreatAsAtomicUnit=on
  Mux : Mux  Inputs=2
  alfa/beta : Outport
  wires:
  abc/1 -> Demux/1
  Demux/2 -> MATLAB Function/2(b)
  MATLAB Function/1(d) -> Mux/1
  Demux/1 -> MATLAB Function/1(a)
  Demux/3 -> MATLAB Function/3(c)
  MATLAB Function/2(e) -> Mux/2
  Mux/1 -> alfa/beta/1

== system Simulacion/Control1/Angulo/abc-->alfa//beta ==
  abc : Inport
  Demux : Demux  Outputs=3
  MATLAB Function : MATLAB Function  TreatAsAtomicUnit=on
  Mux : Mux  Inputs=2
  alfa/beta : Outport
  wires:
  abc/1 -> Demux/1
  Demux/2 -> MATLAB Function/2(b)
  MATLAB Function/1(d) -> Mux/1
  Demux/1 -> MATLAB Function/1(a)
  Demux/3 -> MATLAB Function/3(c)
  MATLAB Function/2(e) -> Mux/2
  Mux/1 -> alfa/beta/1

== matlab function Simulacion/Control1/alfa//beta-->abc/MATLAB Function ==
  data: a input; d output; b input; e output; f output
function [d,e,f] = fcn(a,b)

d=a;
e=-(a/2)+b*(sqrt(3)/2);
f=-(a/2)-b*(sqrt(3)/2);

== matlab function Simulacion/Control1/DQ-->alfa//beta/MATLAB Function ==
  data: a input; d output; b input; e output; c input
function [d,e] = fcn(a,b,c)

d=a*cos(c)+b*sin(c);
e=-a*sin(c)+b*cos(c);

== matlab function Simulacion/Control1/abc-->alfa//beta/MATLAB Function ==
  data: a input; d output; b input; e output; c input
function [d,e] = fcn(a,b,c)

d=2/3*(a-b/2-c/2);
e=2/3*(b*(sqrt(3)/2)-c*(sqrt(3)/2));

== matlab function Simulacion/Control1/d//q-->alfa//beta/MATLAB Function ==
  data: a input; d output; b input; e output; c input
function [d,e] = fcn(a,b,c)

d=a*cos(c)-b*sin(c);
e=a*cos(c)+b*sin(c);

== matlab function Simulacion/Control/d//q-->DQ/MATLAB Function ==
  data: a input; d output; b input; e output; c input
function [d,e] = fcn(a,b,c)

d=a*cos(c)-b*sin(c);
e=a*cos(c)+b*sin(c);

== matlab function Simulacion/Control/DQ-->abc/MATLAB Function ==
  data: a input; d output; b input; e output; f output
function [d,e,f] = fcn(a,b)

d=a;
e=-(a/2)+b*(sqrt(3)/2);
f=-(a/2)-b*(sqrt(3)/2);

== matlab function Simulacion/Control/DQ-->d//q/MATLAB Function ==
  data: a input; d output; b input; e output; c input
function [d,e] = fcn(a,b,c)

d=a*cos(c)+b*sin(c);
e=-a*sin(c)+b*cos(c);

== matlab function Simulacion/Control/abc-->DQ/MATLAB Function ==
  data: a input; d output; b input; e output; c input
function [d,e] = fcn(a,b,c)

d=2/3*(a-b/2-c/2);
e=2/3*(b*(sqrt(3)/2)-c*(sqrt(3)/2));

== matlab function Simulacion/Control/Angulo/abc-->DQ/MATLAB Function ==
  data: a input; d output; b input; e output; c input
function [d,e] = fcn(a,b,c)

d=2/3*(a-b/2-c/2);
e=2/3*(b*(sqrt(3)/2)-c*(sqrt(3)/2));

== matlab function Simulacion/Control/Cancelacion de cc/MATLAB Function ==
  data: a input; g output; b input; h output; c input; d input; e input; f input
function [g,h] = fcn(a,b,c,d,e,f)


Lsi=0.087e-3;                     %Inductancia de fuga (Estator y rotor) (H)
Lm=2.5e-3;                        %Inductancia de magnetizacion (H)
Ls=Lm+Lsi;                        %Inductancia del estator (H)
Lr=Lm+Lsi;                        %Inductancia del rotor (H)
sigma=1-Lm^2/(Ls*Lr);


vsigma=sigma;

g=a-e*vsigma*Lr*d;
h=b+e*vsigma*Lr*c+e*(Lm/Ls)*f;

== matlab function Simulacion/Control1/Angulo/abc-->alfa//beta/MATLAB Function ==
  data: a input; d output; b input; e output; c input
function [d,e] = fcn(a,b,c)

d=2/3*(a-b/2-c/2);
e=2/3*(b*(sqrt(3)/2)-c*(sqrt(3)/2));

== matlab function Simulacion/Control1/Cancelacion de cc/MATLAB Function ==
  data: a input; g output; b input; h output; c input; d input
function [g,h] = fcn(a,b,c,d)

f=50;
Lg=400e-6; 

g=a-d*Lg*(2*pi*f);
h=b-c*Lg*(2*pi*f);
